simulink model "YCrCbWithHSV-NalinSir"  (R2016a)
settings: Solver=VariableStepAuto  StartTime=0.0  StopTime=inf  RelTol=1e-3
undefined symbols (not defined in the file): A, gray, none, Rec, SDTV, videoinput
libraries: visionconversions x4, imaqlib x1, visionsinks x1
settings Model: Creator=Nalin  LastModifiedBy=YASARA

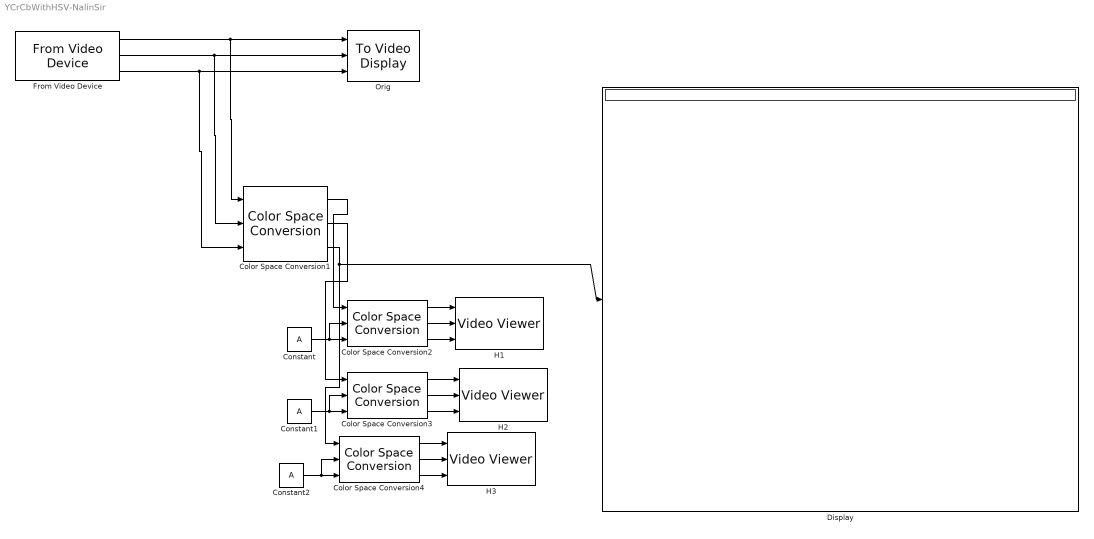
== system YCrCbWithHSV-NalinSir ==
  Color Space Conversion1 : visionconversions/Color Space  Conversion  conversion=Obsolete  conversionActive=R'G'B' to Y'CbCr  wp_str=D65  rec=Rec. 601 (SDTV)  sys=1125/60/2:1  imagePorts=Separate color signals
  Color Space Conversion2 : visionconversions/Color Space  Conversion  conversion=Obsolete  conversionActive=HSV to R'G'B'  wp_str=D65  rec=Rec. 601 (SDTV)  sys=1125/60/2:1  imagePorts=Separate color signals
  Color Space Conversion3 : visionconversions/Color Space  Conversion  conversion=Obsolete  conversionActive=HSV to R'G'B'  wp_str=D65  rec=Rec. 601 (SDTV)  sys=1125/60/2:1  imagePorts=Separate color signals
  Color Space Conversion4 : visionconversions/Color Space  Conversion  conversion=Obsolete  conversionActive=HSV to R'G'B'  wp_str=D65  rec=Rec. 601 (SDTV)  sys=1125/60/2:1  imagePorts=Separate color signals
  Constant : Constant  Value=A  OutDataTypeStr=Inherit: Inherit via back propagation
  Constant1 : Constant  Value=A  OutDataTypeStr=Inherit: Inherit via back propagation
  Constant2 : Constant  Value=A  OutDataTypeStr=Inherit: Inherit via back propagation
  Display : Display
  From Video Device : imaqlib/From Video Device  DeviceMenu=(none)  Device=winvideo 2 (USB Video Device)  ObjConstructor=videoinput('winvideo', 2)  VideoFormatMenu=(none)  VideoFormat=YUY2_640x480  VideoSource=input1  ROIPosition=[0 0 480 640]  EnableHWTrigger=off  TriggerConfiguration=none/none  SampleTime=1/30  OutputPortsMode=Separate color signals  DataType=double  CanDoHWTrigger=no  ReturnedColorSpace=rgb  BlockHandle=434.0011  ROIWidth=640  ROIHeight=480  ROIColumn=0  ROIRow=0  EngXMLPath=C:\Program Files\MATLAB\R2016a\toolbox\imaq\imaq\private  DevXMLPath=C:\Program Files\MATLAB\R2016a\toolbox\imaq\imaqadaptors\win64  EngLibPath=C:\Program Files\MATLAB\R2016a\toolbox\imaq\imaqblks\imaqmex\win64  ColorSpace=rgb  BayerSensorAlignment=grbg
  H1 : VideoViewer  colormapValue=gray(256)  FigPos=[12.2 522 575.2 415.2]
  H2 : VideoViewer  colormapValue=gray(256)  FigPos=[9 848 575 415]
  H3 : VideoViewer  colormapValue=gray(256)  FigPos=[576.2 520.4 575.2 415.2]
  Orig : visionsinks/To Video Display  windowSizeMode=True size (1:1)  openAtMdlStart=on  fullScreen=off  videoWindowX=1119  videoWindowY=112  saveWindowSize=off  videoWindowWidth=640  videoWindowHeight=480  inputColorFormat=RGB  inputType=Obsolete  imagePorts=Separate color signals  OutputDevice=On-screen video monitor  dataOrg=Column-major  isWindowOpen=off
  wires:
  From Video Device/1 -> Color Space Conversion1/1, Orig/1
  From Video Device/2 -> Color Space Conversion1/2, Orig/2
  From Video Device/3 -> Color Space Conversion1/3, Orig/3
  Color Space Conversion1/1 -> Color Space Conversion2/1
  Color Space Conversion1/2 -> Color Space Conversion3/1
  Color Space Conversion1/3 -> Display/1, Color Space Conversion4/1
  Constant/1 -> Color Space Conversion2/2, Color Space Conversion2/3
  Color Space Conversion2/1 -> H1/1
  Color Space Conversion2/2 -> H1/2
  Color Space Conversion2/3 -> H1/3
  Constant1/1 -> Color Space Conversion3/2, Color Space Conversion3/3
  Color Space Conversion3/1 -> H2/1
  Color Space Conversion3/2 -> H2/2
  Color Space Conversion3/3 -> H2/3
  Constant2/1 -> Color Space Conversion4/2, Color Space Conversion4/3
  Color Space Conversion4/1 -> H3/1
  Color Space Conversion4/2 -> H3/2
  Color Space Conversion4/3 -> H3/3
